simulink model "simu"  (R2024b)
settings: Solver=VariableStepAuto  StartTime=0.0  StopTime=3  RelTol=1e-3
values from neighbouring files (symbols this model uses):
  A = [A1, zeros(3) ... (first row only)    [threetank.m]    (also in threetank_identification.m = [-0.011698, 0, 0.011698; threetank_mimo.m = [A1 zeros(size(A1)); zeros(size(A2)) A2])
  B = [B11(2:end), B12(2:end) ... (first row only)    [threetank.m]    (also in threetank_identification.m = [64.9351, 0; threetank_mimo.m = [B1 B2; B3 B4])
  D = [D1, zeros(3,1) ... (first row only)    [threetank.m]    (also in threetank_mimo.m = [D1 zeros(size(D1)); zeros(size(D2)) D2])
  H = [H1, [0, 0, 0] ... (first row only)    [threetank.m]    (also in threetank_mimo.m = [H zeros(size(H)); zeros(size(H)) H])
  KE = K*E    [threetank.m]
  KF = K*F    [threetank.m]
  kr = zeros(2)    [threetank.m]
  Ts = 0.03    [threetank.m]    (also in threetank_identification.m = t(2) - t(1); threetank_mimo.m)
libraries: cstblocks x2
settings Model: Creator=room2  LastModifiedBy=room2

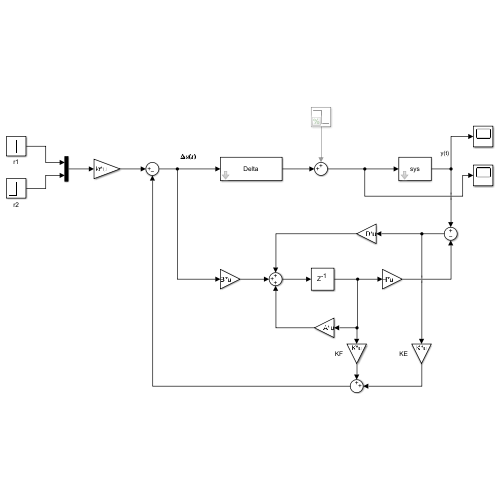
[thumbnail: Simulink's stored preview of the top-level diagram]
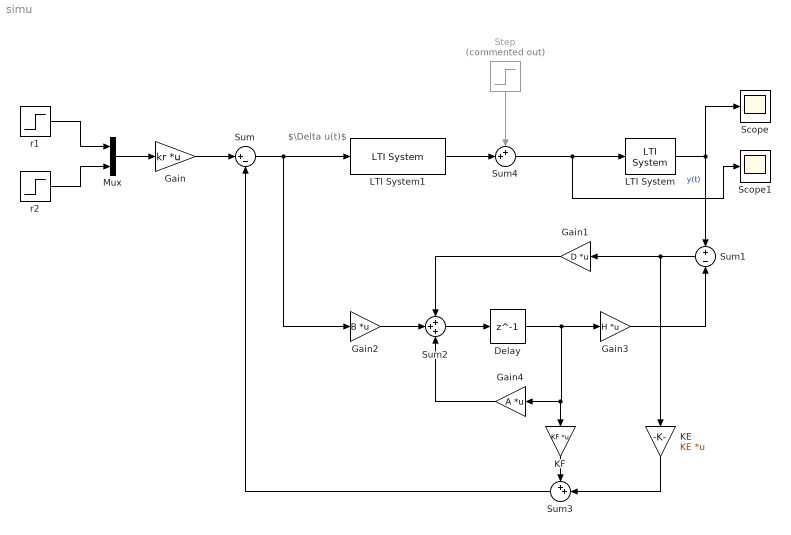
== system simu ==
  note: $\Delta u(t)$
  Delay : Delay  DelayLength=1  SampleTime=Ts
  Gain : Gain  Gain=kr  Multiplication=Matrix(K*u)
  Gain1 : Gain  Gain=D  Multiplication=Matrix(K*u)
  Gain2 : Gain  Gain=B  Multiplication=Matrix(K*u)
  Gain3 : Gain  Gain=H  Multiplication=Matrix(K*u)
  Gain4 : Gain  Gain=A  Multiplication=Matrix(K*u)
  KE : Gain  Gain=KE  Multiplication=Matrix(K*u)
  KF : Gain  Gain=KF  Multiplication=Matrix(K*u)
  LTI System : cstblocks/LTI System  sys=sys  IC=[]  PadeOrder=0
  LTI System1 : cstblocks/LTI System  sys=Delta  IC=[]  PadeOrder=0
  Mux : Mux  Inputs=2
  Scope : Scope
  Scope1 : Scope
  Step : Step  Commented=on  Time=10  After=-1  SampleTime=0
  Sum : Sum  Inputs=|+-
  Sum1 : Sum  Inputs=+|-
  Sum2 : Sum  Inputs=+++
  Sum3 : Sum  Inputs=++|
  Sum4 : Sum  Inputs=++|
  r1 : Step  Time=1.5  Before=0.5  After=0.4  SampleTime=0
  r2 : Step  Time=0  After=0.3  SampleTime=0
  wires:
  Sum2/1 -> Delay/1
  LTI System/1 -> Scope/1, Sum1/1  "y(t)"
  Gain4/1 -> Sum2/3
  Delay/1 -> KF/1, Gain4/1, Gain3/1
  Sum/1 -> Gain2/1, LTI System1/1
  KE/1 -> Sum3/2
  Gain3/1 -> Sum1/2
  Gain/1 -> Sum/1
  Step/1 -> Sum4/1
  LTI System1/1 -> Sum4/2
  Sum3/1 -> Sum/2
  KF/1 -> Sum3/1
  Sum1/1 -> Gain1/1, KE/1
  Gain2/1 -> Sum2/2
  Gain1/1 -> Sum2/1
  r1/1 -> Mux/1
  Mux/1 -> Gain/1
  r2/1 -> Mux/2
  Sum4/1 -> Scope1/1, LTI System/1
